simulink model "Sprung"  (Simulink 7.7)
settings: Solver=ode45  StartTime=0.0  StopTime=9999  RelTol=1e-3
libraries: simulink x1, aerolibatmos2 x1
settings Model: Creator=andreas  LastModifiedBy=andreas

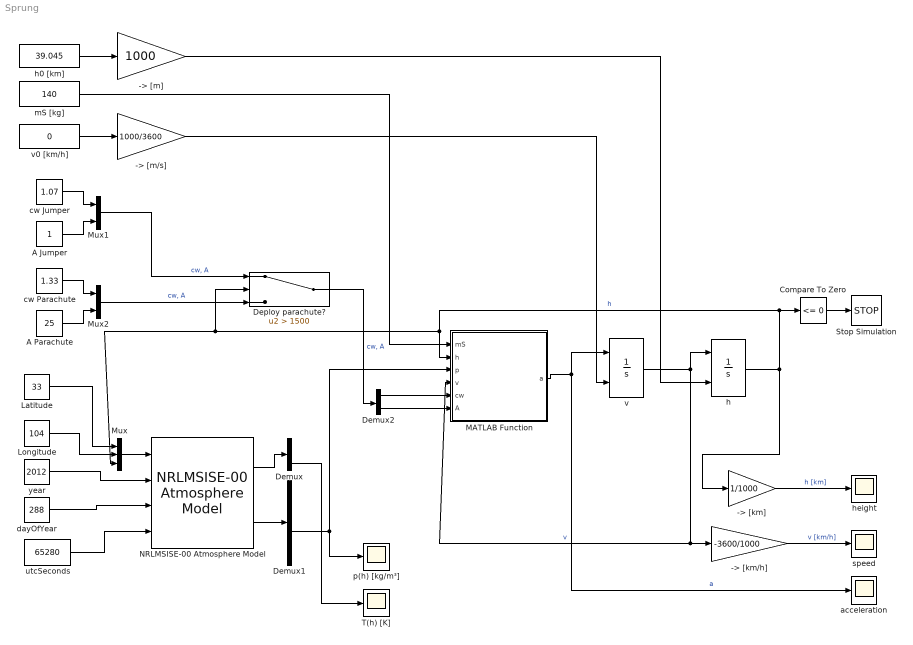
== system Sprung ==
  -> [km/h] : Gain  Gain=-3600/1000
  -> [km] : Gain  Gain=1/1000
  -> [m/s] : Gain  Gain=1000/3600
  -> [m] : Gain  Gain=1000
  A Jumper : Constant
  A Parachute : Constant  Value=25
  Compare To Zero : simulink/Logic and Bit Operations/Compare To Zero  SystemSampleTime=-1  relop=<=  LogicOutDataTypeMode=boolean
  Demux : Demux  Outputs=2
  Demux1 : Demux  Outputs=9
  Demux2 : Demux  Outputs=2
  Deploy parachute? : Switch  Criteria=u2 > Threshold  Threshold=1500
  Latitude : Constant  Value=33
  Longitude : Constant  Value=104
  MATLAB Function : Stateflow chart  TreatAsAtomicUnit=on
  Mux : Mux  Inputs=3
  Mux1 : Mux  Inputs=2
  Mux2 : Mux  Inputs=2
  NRLMSISE-00 Atmosphere Model : aerolibatmos2/NRLMSISE-00 Atmosphere Model  SystemSampleTime=-1  units=Metric (MKS)  lst_input=off  flux_ap_input=off  flags_input=Internal  flags=ones(1,23)  oxygen_in=off  action=Warning
  Stop Simulation : Stop
  T(h) [K] : Scope
      settings: TimeRange=500  YMin=200  YMax=300
  acceleration : Scope
      settings: TimeRange=500  YMin=-50  YMax=300  SaveName=ScopeData4
  cw Jumper : Constant  Value=1.07
  cw Parachute : Constant  Value=1.33
  dayOfYear : Constant  Value=288
  h : Integrator  InitialConditionSource=external
  h0 [km] : Constant  Value=39.045
  height : Scope
      settings: TimeRange=500  YMin=-1.70530256582424e-16  YMax=40  SaveName=ScopeData2
  mS [kg] : Constant  Value=140
  p(h) [kg/m³] : Scope
      settings: TimeRange=500  YMin=0  YMax=1.4
  speed : Scope
      settings: TimeRange=500  YMin=-0  YMax=1400  SaveName=ScopeData3
  utcSeconds : Constant  Value=65280
  v : Integrator  InitialConditionSource=external
  v0 [km/h] : Constant  Value=0
  year : Constant  Value=2012
  wires:
  Latitude/1 -> Mux/1
  Longitude/1 -> Mux/2
  Mux/1 -> NRLMSISE-00 Atmosphere Model/1
  year/1 -> NRLMSISE-00 Atmosphere Model/2
  dayOfYear/1 -> NRLMSISE-00 Atmosphere Model/3
  utcSeconds/1 -> NRLMSISE-00 Atmosphere Model/4
  h/1 -> Compare To Zero/1, MATLAB Function/2(h), Mux/3, Deploy parachute?/2, -> [km]/1  "h"
  NRLMSISE-00 Atmosphere Model/2 -> Demux1/1
  NRLMSISE-00 Atmosphere Model/1 -> Demux/1
  v0 [km/h]/1 -> -> [m/s]/1
  h0 [km]/1 -> -> [m]/1
  Demux/2 -> T(h) [K]/1
  mS [kg]/1 -> MATLAB Function/1(mS)
  MATLAB Function/1(a) -> v/1, acceleration/1  "a"
  Demux1/6 -> MATLAB Function/3(p), p(h) [kg/m³]/1
  -> [m/s]/1 -> v/2
  -> [m]/1 -> h/2
  v/1 -> h/1, MATLAB Function/4(v), -> [km/h]/1  "v"
  Compare To Zero/1 -> Stop Simulation/1
  cw Jumper/1 -> Mux1/1
  A Jumper/1 -> Mux1/2
  Mux1/1 -> Deploy parachute?/1  "cw, A"
  cw Parachute/1 -> Mux2/1
  A Parachute/1 -> Mux2/2
  Mux2/1 -> Deploy parachute?/3  "cw, A"
  Demux2/1 -> MATLAB Function/5(cw)
  Demux2/2 -> MATLAB Function/6(A)
  Deploy parachute?/1 -> Demux2/1  "cw, A"
  -> [km/h]/1 -> speed/1  "v [km/h]"
  -> [km]/1 -> height/1  "h [km]"

== matlab function MATLAB Function ==
  data: mS input double; a output double; h input double; p input double; v input double; cw input double; A input double
function a = beschleunigung(mS, h, p, v, cw, A)
%#codegen

% Erdmasse [kg]
mE=5.9736*10^24;
% Erdradius (Äquator) [m]
rE=6378137;

% Widerstandsfläche
cwA = cw*A;

% Gravitationskonstante [m³/(kg*s²)]
G=66.7384*10^-12;

a=(-G*(mS*mE)/(rE+h)^2 + 0.5*p*v^2*cwA)/mS;
